simulink model "VAB_non_linear_Discrete_function"  (R2019b)
settings: Solver=VariableStepAuto  StartTime=0.0  StopTime=t_end  FixedStep=Ts  RelTol=1e-3
undefined symbols (not defined in the file or in its folder): controllore, m_c_simulazione, phi_iniziale, phi_p_iniziale, phi_p_setpoint, phi_secondo, theta_iniziale, theta_p_iniziale, theta_secondo, Ts
settings Model: Creator=miche  LastModifiedBy=miche

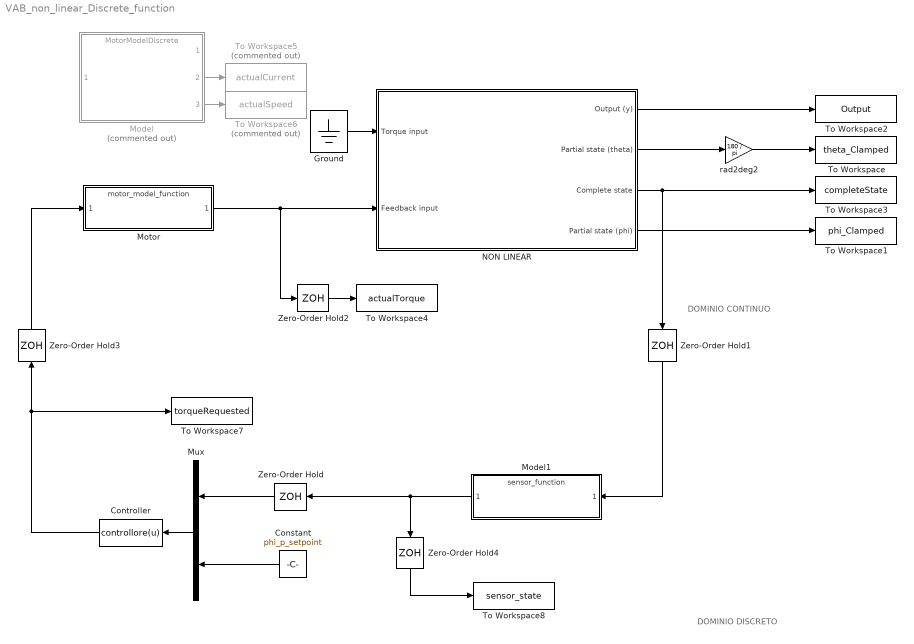
== system VAB_non_linear_Discrete_function ==
  note: DOMINIO DISCRETO
  note: DOMINIO CONTINUO
  Constant : Constant  Value=phi_p_setpoint
  Controller : MATLABFcn  MATLABFcn=controllore(u)
  Ground : Ground
  Model : ModelReference  Commented=on  ModelNameDialog=MotorModelDiscrete.slx  SimulationMode=Normal  ModelReferenceVersion=1.14
  Model1 : ModelReference  ModelNameDialog=sensor_function.slx  SimulationMode=Normal  ModelReferenceVersion=1.1
  Motor : ModelReference  ModelNameDialog=motor_model_function.slx  SimulationMode=Normal  ModelReferenceVersion=1.3
  Mux : Mux  Inputs=2
  NON LINEAR : Subsystem
  To Workspace : ToWorkspace  VariableName=theta_Clamped  SampleTime=-1
  To Workspace1 : ToWorkspace  VariableName=phi_Clamped  SampleTime=-1
  To Workspace2 : ToWorkspace  VariableName=Output  SampleTime=-1
  To Workspace3 : ToWorkspace  VariableName=completeState  SampleTime=-1
  To Workspace4 : ToWorkspace  VariableName=actualTorque  SampleTime=-1
  To Workspace5 : ToWorkspace  Commented=on  VariableName=actualCurrent  SampleTime=-1
  To Workspace6 : ToWorkspace  Commented=on  VariableName=actualSpeed  SampleTime=-1
  To Workspace7 : ToWorkspace  VariableName=torqueRequested  SampleTime=-1
  To Workspace8 : ToWorkspace  VariableName=sensor_state  SampleTime=-1
  Zero-Order Hold{,1..4} (5 alike) : ZeroOrderHold  SampleTime=Ts
  rad2deg2 : Gain  Gain=180 / pi
  wires:
  Constant/1 -> Mux/2
  Zero-Order Hold1/1 -> Model1/1
  Controller/1 -> To Workspace7/1, Zero-Order Hold3/1
  NON LINEAR/1(Output (y)) -> To Workspace2/1
  Zero-Order Hold3/1 -> Motor/1
  Model/3 -> To Workspace6/1
  NON LINEAR/2(Partial state (theta)) -> rad2deg2/1
  Model/2 -> To Workspace5/1
  rad2deg2/1 -> To Workspace/1
  NON LINEAR/4(Partial state (phi)) -> To Workspace1/1
  NON LINEAR/3("Complete state ") -> To Workspace3/1, Zero-Order Hold1/1
  Motor/1 -> Zero-Order Hold2/1, NON LINEAR/2(Feedback input)
  Ground/1 -> NON LINEAR/1(Torque input)
  Zero-Order Hold/1 -> Mux/1
  Zero-Order Hold2/1 -> To Workspace4/1
  Mux/1 -> Controller/1
  Zero-Order Hold4/1 -> To Workspace8/1
  Model1/1 -> Zero-Order Hold4/1, Zero-Order Hold/1

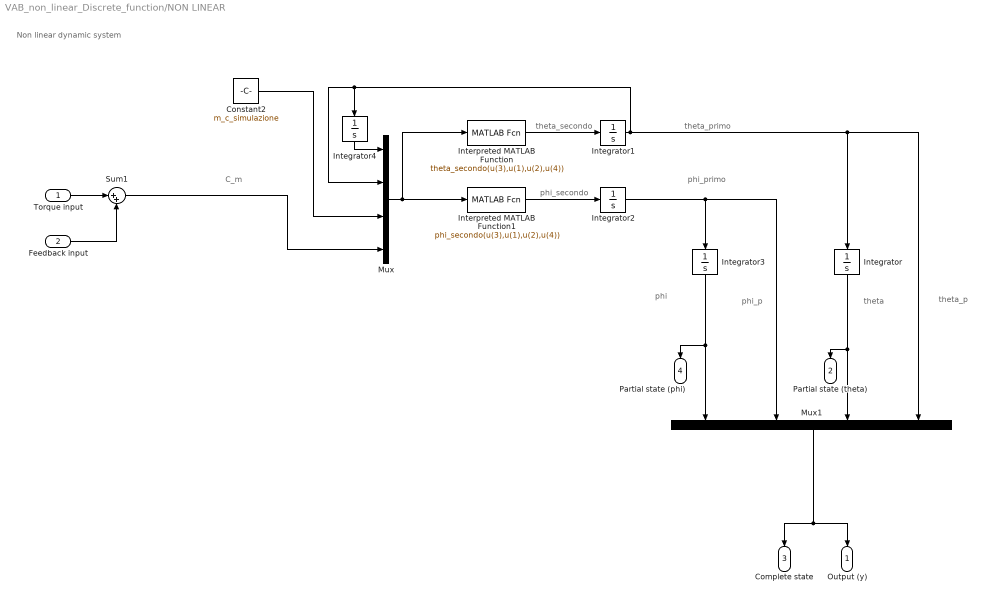
== system VAB_non_linear_Discrete_function/NON LINEAR ==
  note: Non linear dynamic system
  note: phi_primo
  note: phi
  note: theta_p
  note: theta
  note: phi_p
  note: phi_secondo
  note: C_m
  note: theta_secondo
  note: theta_primo
  Torque input : Inport  PortDimensions=1
  Feedback input : Inport  Port=2  PortDimensions=1
  Constant2 : Constant  Value=m_c_simulazione
  Integrator : Integrator  InitialCondition=theta_iniziale
  Integrator1 : Integrator  InitialCondition=theta_p_iniziale  UpperSaturationLimit=100  LowerSaturationLimit=-100
  Integrator2 : Integrator  InitialCondition=phi_p_iniziale
  Integrator3 : Integrator  InitialCondition=phi_iniziale
  Integrator4 : Integrator  InitialCondition=theta_iniziale
  Interpreted MATLAB Function : MATLABFcn  MATLABFcn=theta_secondo(u(3),u(1),u(2),u(4))  OutputDimensions=1
  Interpreted MATLAB Function1 : MATLABFcn  MATLABFcn=phi_secondo(u(3),u(1),u(2),u(4))  OutputDimensions=1
  Mux : Mux
      settings: DisplayOption=signals
  Mux1 : Mux
  Sum1 : Sum  Inputs=|++
  Output (y) : Outport
  Partial state (theta) : Outport  Port=2
  "Complete state " : Outport  Port=3
  Partial state (phi) : Outport  Port=4
  wires:
  Feedback input/1 -> Sum1/2
  Torque input/1 -> Sum1/1
  Integrator3/1 -> Partial state (phi)/1, Mux1/1
  Constant2/1 -> Mux/3
  Sum1/1 -> Mux/4
  Integrator4/1 -> Mux/1
  Interpreted MATLAB Function1/1 -> Integrator2/1
  Integrator2/1 -> Mux1/2, Integrator3/1
  Integrator1/1 -> Integrator4/1, Mux/2, Mux1/4, Integrator/1
  Integrator/1 -> Partial state (theta)/1, Mux1/3
  Interpreted MATLAB Function/1 -> Integrator1/1
  Mux1/1 -> Output (y)/1, "Complete state "/1
  Mux/1 -> Interpreted MATLAB Function/1, Interpreted MATLAB Function1/1
